simulink model "ass6q9"  (R2018a)
settings: Solver=VariableStepAuto  StartTime=0.0  StopTime=10.0  RelTol=1e-3
settings Model: Creator=arjun  LastModifiedBy=arjun

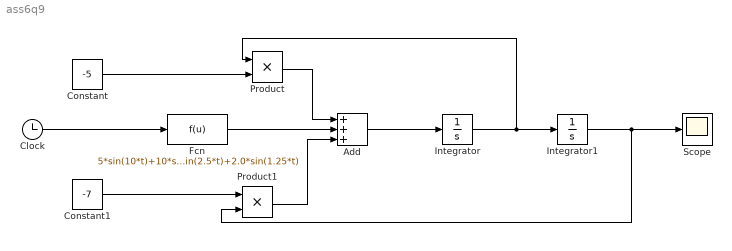
== system ass6q9 ==
  Add : Sum  Inputs=+++
  Clock : Clock
  Constant : Constant  Value=-5
  Constant1 : Constant  Value=-7
  Fcn : Fcn  Expr=5*sin(10*t)+10*sin(5*t)+1.5*sin(2.5*t)+2.0*sin(1.25*t)
  Integrator : Integrator
  Integrator1 : Integrator
  Product : Product
  Product1 : Product
  Scope : Scope
  wires:
  Clock/1 -> Fcn/1
  Fcn/1 -> Add/2
  Constant/1 -> Product/2
  Product/1 -> Add/1
  Constant1/1 -> Product1/1
  Product1/1 -> Add/3
  Add/1 -> Integrator/1
  Integrator/1 -> Product/1, Integrator1/1
  Integrator1/1 -> Product1/2, Scope/1
